simulink model "dfex"  (Simulink 8.5)
settings: Solver=ode45  SolverMode=SingleTasking  StartTime=0.0  StopTime=0.06  RelTol=1e-3  AbsTol=1e-6
libraries: elements x1
settings Model: Creator=PC  LastModifiedBy=PC
settings DataIOCC: LimitDataPoints=off  SaveOutput=off  SaveTime=off
settings OptimizationCC: BlockReduction=off  BooleanDataType=off  ExpressionDepthLimit=128
settings DebuggingCC: SaveWithParameterizedLinksMsg=none  SignalResolutionControl=TryResolveAllWithWarning  MultiTaskDSMMsg=warning  MultiTaskCondExecSysMsg=none  FcnCallInpInsideContextMsg=EnableAllAsError  StateNameClashWarn=none
settings HardwareCC: TargetUnknown=on
settings RTWCC: TemplateMakefile=grt_vc.tmf

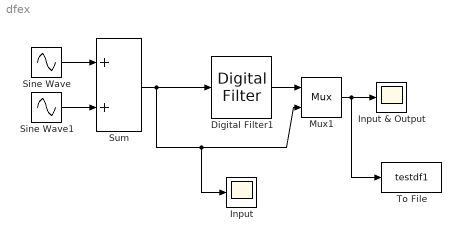
== system dfex ==
  Digital Filter1 : elements/Digital Filter  FilterType=Fourier_Sine  PassType=highpass  IIROrder=3  fs=20*60  CutFre=[180]  DataWindow=20  winsize=1  frequency0=60  FreeZformNum="[0  1 ]"  FreeZformDen=[ 1 ]
  Input : Scope
      settings: TickLabels=on  TimeRange=0.06  YMin=-3  YMax=3
  Input & Output : Scope
      settings: TickLabels=on  TimeRange=0.06  YMin=-2  YMax=2
  Mux1 : Mux  Inputs=2
  Sine Wave : Sin  Frequency=60*2*pi  SampleTime=1/1200
  Sine Wave1 : Sin  Frequency=2*60*2*pi  SampleTime=1/1200
  Sum : Sum  SaturateOnIntegerOverflow=on  InputSameDT=on  OutDataTypeStr=Inherit: Same as first input
  To File : ToFile  Filename=testdf1  MatrixName=testdf1
  wires:
  Mux1/1 -> To File/1, Input & Output/1
  Sine Wave1/1 -> Sum/2
  Sum/1 -> Digital Filter1/1, Input/1, Mux1/2
  Sine Wave/1 -> Sum/1
  Digital Filter1/1 -> Mux1/1
